simulink model "OpenControl"  (Simulink 9.2)
settings: Solver=FixedStepAuto  StartTime=0.0  StopTime=inf  RelTol=1e-3
settings Model: Creator=Dephy Inc  LastModifiedBy=dan
settings DataIOCC: LimitDataPoints=off  SaveFormat=Dataset  SignalLoggingSaveFormat=Dataset
settings OptimizationCC: LifeSpan=auto
settings DebuggingCC: UnderspecifiedInitializationDetection=Simplified  MergeDetectMultiDrivingBlocksExec=error  FcnCallInpInsideContextMsg=error  StateNameClashWarn=none  SFUnexpectedBacktrackingDiag=error  SFNoUnconditionalDefaultTransitionDiag=error  SFExecutionAtInitializationDiag=warning
settings HardwareCC: ProdBitPerPointer=64  ProdBitPerSizeT=64  ProdBitPerPtrDiffT=64  ProdLargestAtomicFloat=Float  ProdIntDivRoundTo=Zero  ProdEndianess=LittleEndian  ProdWordSize=64  ProdHWDeviceType=Intel->x86-64 (Windows64)
settings ModelReferenceCC: PropagateSignalLabelsOutOfModel=on
settings SFSimCC: SimUseLocalCustomCode=on
settings RTWCC: RTWUseLocalCustomCode=on
settings CodeAppCC: StateflowObjectComments=off
settings GRTTargetCC: TargetLangStandard=C99 (ISO)  GeneratePreprocessorConditionals=Use local settings  CombineOutputUpdateFcns=on  GRTInterface=off
settings ConfigComp: CovMetricSettings=dwe  CovHtmlReporting=off  CovSaveCumulativeToWorkspaceVar=off  CovSaveSingleToWorkspaceVar=off  CovExternalEMLEnable=on

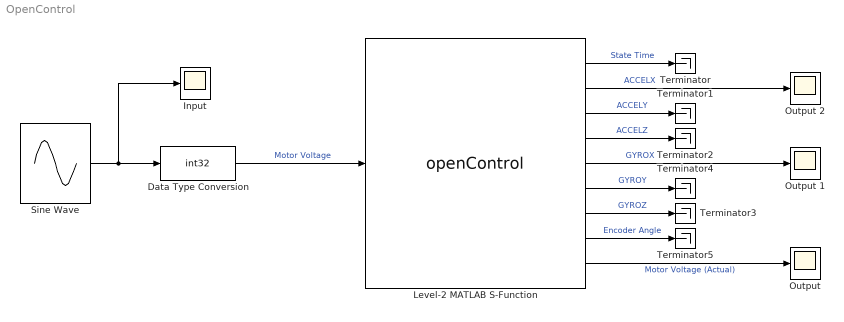
== system OpenControl ==
  Data Type Conversion : DataTypeConversion  OutDataTypeStr=int32
  Input : Scope
  Level-2 MATLAB S-Function : M-S-Function  FunctionName=openControl
  Output : Scope
  Output 1 : Scope
  Output 2 : Scope
  Sine Wave : Sin  Amplitude=1000  Bias=2000  Frequency=0.07  SampleTime=0
  Terminator{,1..5} (6 alike) : Terminator
  wires:
  Data Type Conversion/1 -> Level-2 MATLAB S-Function/1  "Motor Voltage"
  Sine Wave/1 -> Input/1, Data Type Conversion/1
  Level-2 MATLAB S-Function/9 -> Output/1  "Motor Voltage (Actual)"
  Level-2 MATLAB S-Function/2 -> Output 2/1  "ACCELX"
  Level-2 MATLAB S-Function/5 -> Output 1/1  "GYROX"
  Level-2 MATLAB S-Function/1 -> Terminator/1  "State Time"
  Level-2 MATLAB S-Function/4 -> Terminator2/1  "ACCELZ"
  Level-2 MATLAB S-Function/3 -> Terminator1/1  "ACCELY"
  Level-2 MATLAB S-Function/8 -> Terminator5/1  "Encoder Angle"
  Level-2 MATLAB S-Function/7 -> Terminator3/1  "GYROZ"
  Level-2 MATLAB S-Function/6 -> Terminator4/1  "GYROY"
